simulink model "SimscapeSystemLevel_e8_IPMSM_HWJandVent_ROM"  (R2021b)
settings: Solver=VariableStepAuto  StartTime=0.0  StopTime=300  FixedStep=1  RelTol=1e-3  AbsTol=1e-3
model workspace (MAT data in the model file):
  AdjacencyMat = [0 0 0 0 0 0 0 0 0 0 0 0 ... (15129 elements, 123x123)]
  CapMat = [1e+20 2196.70091586 387.653102799 193.8265514 1962.34710525 387.653102799 193.8265514 1962.34710525 1266.59353814 268.053957132 416.539515956 175.715078 ... (123 elements, 123x1)]
  CoolantArrayIdxs = [20 21 22 23 24 25 26 27 35 36 37 84 ... (19 elements, 19x1)]
  Friction_Loss_Mat = [0 0 0 0 0 0 0 0 0 0 0 0 ... (2340 elements, 39x60)]
  InletCoolIdxs = [37; 38]
  Iron_Loss_Rotor_Back_Iron_Mat = [0.0117705351991 0.0198175800092 0.0246057415963 0.0256631766661 0.0240576767285 0.0207771722396 0.0168311502834 0.0133395315761 0.0115512535049 0.0120779527774 0.0143067244388 0.0171516443454 ... (2340 elements, 39x60)]
  Iron_Loss_Rotor_Pole_Mat = [1.45649756865 1.4525095653 1.42942652973 1.39109338754 1.34251579982 1.287439524 1.22885659237 1.16930852698 1.11098912611 1.05484046499 0.999976047808 0.944563732162 ... (2340 elements, 39x60)]
  Iron_Loss_Rotor_Tooth_Mat = [0 0 0 0 0 0 0 0 0 0 0 0 ... (2340 elements, 39x60)]
  Iron_Loss_Stator_Back_Iron_Mat = [38.5419456951 37.774471759 36.7837540443 35.6885758764 34.5272571596 33.3324529178 32.136302555 30.9744032473 29.8863152048 28.8790573391 27.8876077961 26.8074662049 ... (2340 elements, 39x60)]
  Iron_Loss_Stator_Tooth_Mat = [42.0610884508 41.0604961882 40.1804594162 39.4285940164 38.704339026 37.9602455604 37.1844153901 36.3902226975 35.6050856075 34.8287218867 34.0007237809 33.0439458619 ... (2340 elements, 39x60)]
  LossDistrForEachType = [0 0 0 0 0 0 0 0 0 0 0 0 ... (1968 elements, 16x123)]
  Magnet_Loss_Mat = [0.0995193918038 0.0928899922278 0.0868628846748 0.0818830115456 0.0774722500184 0.0732395922727 0.0687988836096 0.0636930921801 0.0573503948699 0.0496000064543 0.0410757743485 0.0326817704515 ... (2340 elements, 39x60)]
  OutletCoolIdxs = [20; 107]
  ResMat = [0 2.49009256841 6.64572241429 1000000000 1.39790968864 6.64402802995 1000000000 1.39156082742 1000000000 1000000000 1000000000 1000000000 ... (15129 elements, 123x123)]
  RotorCopperTempCoefResistivity = 0.00393
  Rotor_Cage_Loss_Mat = [0 0 0 0 0 0 0 0 0 0 0 0 ... (2340 elements, 39x60)]
  ShaftTorqueVec = [-287.262157301 -272.268610731 -257.275064161 -242.281517591 -227.287971021 -212.294424451 -197.300877881 -182.307331311 -167.31378474 -152.32023817 -137.3266916 -122.33314503 ... (39 elements, 1x39)]
  SpeedVec = [500 661.016949153 822.033898305 983.050847458 1144.06779661 1305.08474576 1466.10169492 1627.11864407 1788.13559322 1949.15254237 2110.16949153 2271.18644068 ... (60 elements, 1x60)]
  StateSpaceND : object (value not decoded)
  StatorCopperTempCoefResistivity = 0.00393
  Stator_Copper_Loss_Mat = [3925.33912093 3510.19452231 3089.33767218 2711.80000483 2370.99356953 2062.06508217 1781.35176729 1526.02799256 1293.87708125 1083.15658499 892.54525431 720.809889245 ... (2340 elements, 39x60)]
  Stray_Load_Loss_Mat = [0 0 0 0 0 0 0 0 0 0 0 0 ... (2340 elements, 39x60)]
  Stray_Loss_Stator_Iron_Proportion = 0.95
  Tgiven = 20
  TnodesInit = [25 25 25 25 25 25 25 25 25 25 25 25 ... (123 elements, 123x1)]
  TrefRotor = 20
  TrefStator = 20
  Windage_Loss_Mat = [0 0 0 0 0 0 0 0 0 0 0 0 ... (2340 elements, 39x60)]
libraries: fl_lib x33, nesl_utility x13, mcadROM_lib x4, simulink_extras x2, autolibshared x1, slpidlib x1, SimscapeFluids_lib x1
(part 2 of 2)

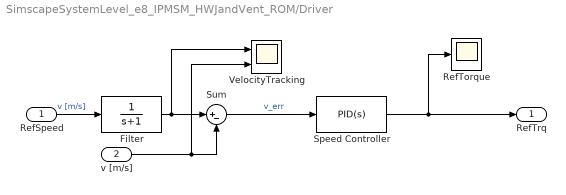
== system SimscapeSystemLevel_e8_IPMSM_HWJandVent_ROM/Driver ==
  RefSpeed : Inport
  v [m/s] : Inport  Port=2
  Filter : TransferFcn  Denominator=[1 1]
  RefTorque : Scope
  Speed Controller : slpidlib/PID Controller  Controller=PID  Form=Parallel  TimeDomain=Continuous-time  UseExternalTs=off  SampleTime=-1  IntegratorMethod=Forward Euler  FilterMethod=Forward Euler  ControllerParametersSource=internal  P=50  I=1e-1  D=0  UseFilter=on  N=100  TunerSelectOption=Transfer Function Based (PID Tuner App)  InitialConditionSource=internal  InitialConditionForIntegrator=0  InitialConditionForFilter=0  DifferentiatorICPrevScaledInput=0  ExternalReset=none  TrackingMode=off  Kt=1  LimitOutput=on  SatLimitsSource=internal  UpperSaturationLimit=150  LowerSaturationLimit=-150  LinearizeAsGain=on  AntiWindupMode=none  Kb=1  POutMin=[]  POutMax=[]  IOutMin=[]  IOutMax=[]  DOutMin=[]  DOutMax=[]  NOutMin=[]  NOutMax=[]  SumOutMin=[]  SumOutMax=[]  SaturationOutMin=[]  SaturationOutMax=[]  PParamMin=[]  PParamMax=[]  IParamMin=[]  IParamMax=[]  DParamMin=[]  DParamMax=[]  NParamMin=[]  NParamMax=[]  KbParamMin=[]  KbParamMax=[]  KtParamMin=[]  KtParamMax=[]  KbOutMin=[]  KbOutMax=[]  KtOutMin=[]  KtOutMax=[]  IntegratorOutMin=[]  IntegratorOutMax=[]  FilterOutMin=[]  FilterOutMax=[]  SumI1OutMin=[]  SumI1OutMax=[]  SumI2OutMin=[]  SumI2OutMax=[]  SumI3OutMin=[]  SumI3OutMax=[]  SumI4OutMin=[]  SumI4OutMax=[]  SumDOutMin=[]  SumDOutMax=[]  DifferentiatorOutMin=[]  DifferentiatorOutMax=[]  FilterDiffOutCoefMin=[]  FilterDiffOutCoefMax=[]  ReciprocalOutMin=[]  ReciprocalOutMax=[]  SumDenOutMin=[]  SumDenOutMax=[]  SumNumOutMin=[]  SumNumOutMax=[]  DivideOutMin=[]  DivideOutMax=[]  UdiffTsProdOutMin=[]  UdiffTsProdOutMax=[]  NTsProdOutMin=[]  NTsProdOutMax=[]  UintegralTsProdOutMin=[]  UintegralTsProdOutMax=[]  UngainTsProdOutMin=[]  UngainTsProdOutMax=[]  FilterDenConstantOutDataTypeStr=Inherit: Inherit via back propagation  FilterDenConstantOutMin=[]  FilterDenConstantOutMax=[]  PCopyOutDataTypeStr=Inherit: Inherit via back propagation  PCopyOutMin=[]  PCopyOutMax=[]  NCopyOutDataTypeStr=Inherit: Inherit via back propagation  NCopyOutMin=[]  NCopyOutMax=[]  IntegratorContinuousStateAttributes=''  IntegratorStateMustResolveToSignalObject=off  IntegratorRTWStateStorageClass=Auto  FilterContinuousStateAttributes=''  FilterStateMustResolveToSignalObject=off  FilterRTWStateStorageClass=Auto  ParallelPVariant=InternalParameters  IdealPVariant=Disabled  IVariant=InternalParameters  DVariant=InternalParameters  IntegratorVariant=Continuous  SatVariant=Enabled  AWVariant=Passthrough  PCopyVariant=Disabled  TRVariant=Disabled  FdbkBlocksVariant=Forward  IdealPFdbkVariant=Disabled  SatFdbkVariant=Disabled  DerivativeFilterVariant=ContFilter  NVariant=InternalParameters  NCopyVariant=Disabled  FilterICVariant=InternalICsFilter  IntegratorICVariant=InternalICs  ExternalResetVariant=Disabled  TRSumVariant=Passthrough  SumFdbkVariant=Disabled  SumVariant=Sum_PID  TsampFilterVariant=InternalTs  TsampNgainVariant=Passthrough  TsampIntegralVariant=Passthrough  ExternalSaturationOutDataTypeStr=Inherit: Same as second input
  Sum : Sum  Inputs=|+-
  VelocityTracking : Scope  NumInputPorts=2
  RefTrq : Outport
  wires:
  v [m/s]/1 -> VelocityTracking/2, Sum/2
  Sum/1 -> Speed Controller/1  "v_err"
  Speed Controller/1 -> RefTorque/1, RefTrq/1
  RefSpeed/1 -> Filter/1  "v [m/s]"
  Filter/1 -> VelocityTracking/1, Sum/1

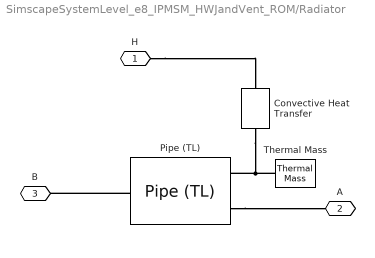
== system SimscapeSystemLevel_e8_IPMSM_HWJandVent_ROM/Radiator ==
  Convective Heat Transfer : fl_lib/Thermal/Thermal Elements/Convective Heat Transfer  area=5 m^2  heat_tr_coeff=20 W/(m^2*K)  T_specify=off  T_priority=None  T=0 K  T_nominal_specify=off  T_nominal_unit=K  T_nominal_value=1  Q_specify=off  Q_priority=None  Q=0 W  Q_nominal_specify=off  Q_nominal_unit=W  Q_nominal_value=1
  Pipe (TL) : fl_lib/Thermal Liquid/Elements/Pipe (TL)  length=5 m  area=0.01 m^2  Dh=0.1128 m  length_add=1 m  roughness=15e-6 m  Re_lam=2000  Re_tur=4000  shape_factor=64  Nu_lam=3.66  dynamic_compressibility=simscape.enum.onoff.on  inertia=simscape.enum.onoff.off  p0=0.101325 MPa  T0=TnodesInit(1) degC  mdot0=0 kg/s
      settings: SourceProductBaseCode=SS
  Thermal Mass : fl_lib/Thermal/Thermal Elements/Thermal Mass  mass=3 kg  sp_heat=447 J/(K*kg)  T_specify=on  T_priority=High  T=TnodesInit(1) degC  T_nominal_specify=off  T_nominal_unit=K  T_nominal_value=1  Q_specify=off  Q_priority=None  Q=0 W  Q_nominal_specify=off  Q_nominal_unit=W  Q_nominal_value=1
  H : PMIOPort  Side=Left
  A : PMIOPort  Port=2  Side=Left
  B : PMIOPort  Port=3  Side=Right
  connections:
  Thermal Mass/LConn1 -- Convective Heat Transfer/LConn1 -- Pipe (TL)/LConn2
  Pipe (TL)/LConn1 -- A/RConn1
  Pipe (TL)/RConn1 -- B/RConn1
  H/RConn1 -- Convective Heat Transfer/RConn1

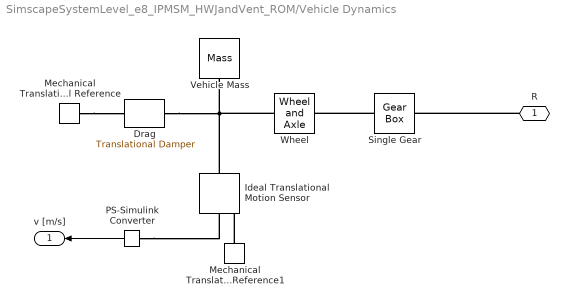
== system SimscapeSystemLevel_e8_IPMSM_HWJandVent_ROM/Vehicle Dynamics ==
  Drag : fl_lib/Mechanical/Translational Elements/Translational Damper  D=25 N/(m/s)  v_specify=off  v_priority=None  v=0 m/s  v_nominal_specify=off  v_nominal_unit=m/s  v_nominal_value=1  f_specify=off  f_priority=None  f=0 N  f_nominal_specify=off  f_nominal_unit=N  f_nominal_value=1
  Ideal Translational Motion Sensor : fl_lib/Mechanical/Mechanical Sensors/Ideal Translational Motion Sensor  offset=0 m
  Mechanical Translational Reference : fl_lib/Mechanical/Translational Elements/Mechanical Translational Reference
  Mechanical Translational Reference1 : fl_lib/Mechanical/Translational Elements/Mechanical Translational Reference
  PS-Simulink Converter : nesl_utility/PS-Simulink Converter  PhysicalDomain=network_engine_domain  SubClassName=ps_output  LeftPortType=input  RightPortType=output  PseudoPeriodic=off  Frequencies=[]  Unit=m/s  AffineConversion=off
      settings: SourceProductBaseCode=PW,SS
  Single Gear : fl_lib/Mechanical/Mechanisms/Gear Box  ratio=1/5  t_in_specify=off  t_in_priority=None  t_in=0 N*m  t_in_nominal_specify=off  t_in_nominal_unit=N*m  t_in_nominal_value=1  t_out_specify=off  t_out_priority=None  t_out=0 N*m  t_out_nominal_specify=off  t_out_nominal_unit=N*m  t_out_nominal_value=1
  Vehicle Mass : fl_lib/Mechanical/Translational Elements/Mass  mass=2000 kg  num_ports=foundation.enum.numPorts2.one  v_specify=off  v_priority=High  v=0 m/s  v_nominal_specify=off  v_nominal_unit=m/s  v_nominal_value=1  f_specify=off  f_priority=None  f=0 N  f_nominal_specify=off  f_nominal_unit=N  f_nominal_value=1
  Wheel : fl_lib/Mechanical/Mechanisms/Wheel and Axle  R=0.15 m  or=1  t_specify=off  t_priority=None  t=0 N*m  t_nominal_specify=off  t_nominal_unit=N*m  t_nominal_value=1  f_specify=off  f_priority=None  f=0 N  f_nominal_specify=off  f_nominal_unit=N  f_nominal_value=1
  R : PMIOPort  Side=Right
  v [m/s] : Outport
  wires:
  PS-Simulink Converter/1 -> v [m/s]/1
  connections:
  R/RConn1 -- Single Gear/RConn1
  Single Gear/LConn1 -- Wheel/LConn1
  Wheel/RConn1 -- Ideal Translational Motion Sensor/LConn1 -- Drag/LConn1 -- Vehicle Mass/LConn1
  Mechanical Translational Reference/LConn1 -- Drag/RConn1
  Mechanical Translational Reference1/LConn1 -- Ideal Translational Motion Sensor/RConn1
  PS-Simulink Converter/LConn1 -- Ideal Translational Motion Sensor/RConn2

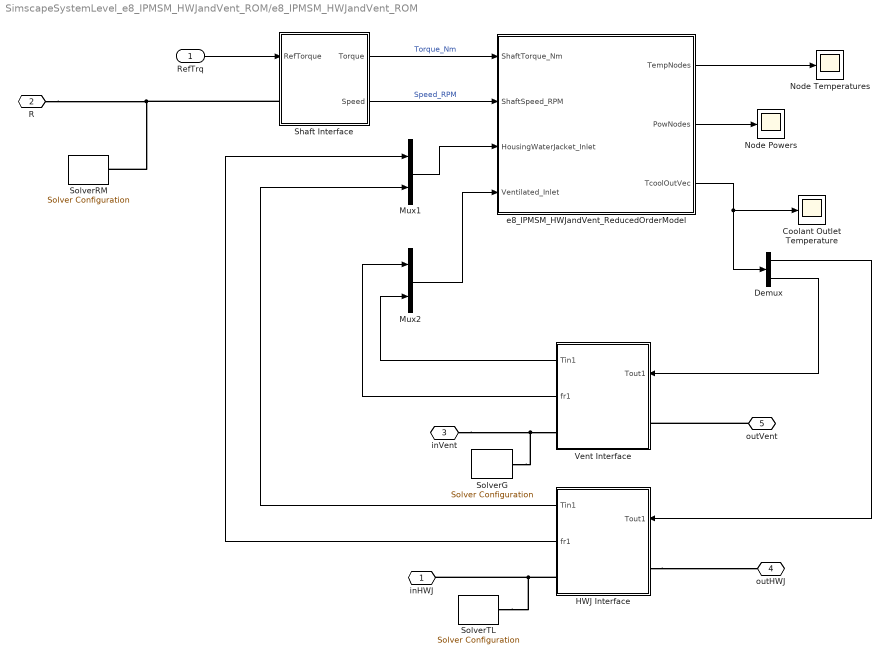
== system SimscapeSystemLevel_e8_IPMSM_HWJandVent_ROM/e8_IPMSM_HWJandVent_ROM ==
  RefTrq : Inport
  Coolant Outlet Temperature : Scope
  Demux : Demux  Outputs=2
  HWJ Interface : Subsystem
      settings: PortSchema="{\"entries\":[{\"content\":{\"sides\":[{\"content\":{\"connectorIds\":[\"Out1\",\"Out2\",\"LConn1\"]},\"type\":\"ConnectorPlacement.EquallySpacedRectSide\",\"uuid\":\"a0734607-c8e3-4baa-99d0-f684b459279a\"},{\"content\":{\"connectorIds\":[\"In1\",\"RConn1\"],\"side\":\"RIGHT\"},\"type\":\"ConnectorPlacement.EquallySpacedRectSide\",\"uuid\":\"b656feb5-3093-4bd9-8bf1-21827cdeeded\"},{\"content\":{\"connectorIds\":[],\"side\":\"TOP\"},\"type\":\"ConnectorPlacement.EquallySpacedRectSide\",\"uuid\":\"2d3f104c-c7aa-4510-969a-a40e5e879ab2\"}]},\"type\":\"ConnectorPlacement.EquallySpacedConnector\",\"uuid\":\"1033d5d5-dd4a-4fd0-a709-c87184322d51\"}],\"packageUris\":[\"http://schema.mathworks.com/mf0/Connector/R2020b\"],\"version\":\"1.0\"}"
  Mux1 : Mux  Inputs=2
  Mux2 : Mux  Inputs=2
  Node Powers : Scope
  Node Temperatures : Scope
  Shaft Interface : Subsystem
  SolverG : nesl_utility/Solver Configuration  PhysicalDomain=network_engine_domain  SubClassName=solver  LeftPortType=input  RightPortType=generic  Tones=[]  Harmonics=[]  SimulateNoise=off  Profile=off  UseLocalSampling=off  EnableSwitchedLinearOptims=on  FrequencyDomain=off  UseCCode=off  RelTol=0.001  AbsTol=1e-06  MinStep=1e-09  ToWorkspace=off  RevertToSquareIcSolve=off  NumHomotopyIterations=100  PhasorMode=off  PhasorModeNumHarmonics=1  DoDC=off  ResidualTolerance=1e-09  UseLocalSolver=off  LocalSolverChoice=NE_BACKWARD_EULER_ADVANCER  LocalSolverSampleTime=0.001  DoFixedCost=off  MaxNonlinIter=3  MaxModeIter=2  ComputeImpulses=off  ImpulseIterations=2  LinearAlgebra=auto  EquationFormulation=NE_TIME_EF  DelaysMemoryBudget=1024  AutomaticFiltering=on  FilteringTimeConstant=0.001  PartitionStorageMethod=AS_NEEDED  PartitionMemoryBudget=1024  PartitionMethod=ROBUST
      settings: SourceProductBaseCode=PW,SS
  SolverRM : nesl_utility/Solver Configuration  PhysicalDomain=network_engine_domain  SubClassName=solver  LeftPortType=input  RightPortType=generic  Tones=[]  Harmonics=[]  SimulateNoise=off  Profile=off  UseLocalSampling=off  EnableSwitchedLinearOptims=on  FrequencyDomain=off  UseCCode=off  RelTol=0.001  AbsTol=1e-06  MinStep=1e-09  ToWorkspace=off  RevertToSquareIcSolve=off  NumHomotopyIterations=100  PhasorMode=off  PhasorModeNumHarmonics=1  DoDC=off  ResidualTolerance=1e-09  UseLocalSolver=off  LocalSolverChoice=NE_BACKWARD_EULER_ADVANCER  LocalSolverSampleTime=0.001  DoFixedCost=off  MaxNonlinIter=3  MaxModeIter=2  ComputeImpulses=off  ImpulseIterations=2  LinearAlgebra=auto  EquationFormulation=NE_TIME_EF  DelaysMemoryBudget=1024  AutomaticFiltering=on  FilteringTimeConstant=0.001  PartitionStorageMethod=AS_NEEDED  PartitionMemoryBudget=1024  PartitionMethod=ROBUST
      settings: SourceProductBaseCode=PW,SS
  SolverTL : nesl_utility/Solver Configuration  PhysicalDomain=network_engine_domain  SubClassName=solver  LeftPortType=input  RightPortType=generic  Tones=[]  Harmonics=[]  SimulateNoise=off  Profile=off  UseLocalSampling=off  EnableSwitchedLinearOptims=on  FrequencyDomain=off  UseCCode=off  RelTol=0.001  AbsTol=1e-06  MinStep=1e-09  ToWorkspace=off  RevertToSquareIcSolve=off  NumHomotopyIterations=100  PhasorMode=off  PhasorModeNumHarmonics=1  DoDC=off  ResidualTolerance=1e-09  UseLocalSolver=off  LocalSolverChoice=NE_BACKWARD_EULER_ADVANCER  LocalSolverSampleTime=0.001  DoFixedCost=off  MaxNonlinIter=3  MaxModeIter=2  ComputeImpulses=off  ImpulseIterations=2  LinearAlgebra=auto  EquationFormulation=NE_TIME_EF  DelaysMemoryBudget=1024  AutomaticFiltering=on  FilteringTimeConstant=0.001  PartitionStorageMethod=AS_NEEDED  PartitionMemoryBudget=1024  PartitionMethod=ROBUST
      settings: SourceProductBaseCode=PW,SS
  Vent Interface : Subsystem
      settings: PortSchema="{\"entries\":[{\"content\":{\"sides\":[{\"content\":{\"connectorIds\":[\"Out1\",\"Out2\",\"LConn1\"]},\"type\":\"ConnectorPlacement.EquallySpacedRectSide\",\"uuid\":\"a0734607-c8e3-4baa-99d0-f684b459279a\"},{\"content\":{\"connectorIds\":[\"In1\",\"RConn1\"],\"side\":\"RIGHT\"},\"type\":\"ConnectorPlacement.EquallySpacedRectSide\",\"uuid\":\"b656feb5-3093-4bd9-8bf1-21827cdeeded\"},{\"content\":{\"connectorIds\":[],\"side\":\"TOP\"},\"type\":\"ConnectorPlacement.EquallySpacedRectSide\",\"uuid\":\"2d3f104c-c7aa-4510-969a-a40e5e879ab2\"}]},\"type\":\"ConnectorPlacement.EquallySpacedConnector\",\"uuid\":\"1033d5d5-dd4a-4fd0-a709-c87184322d51\"}],\"packageUris\":[\"http://schema.mathworks.com/mf0/Connector/R2020b\"],\"version\":\"1.0\"}"
  e8_IPMSM_HWJandVent_ReducedOrderModel : Subsystem
  inHWJ : PMIOPort  Side=Left
  R : PMIOPort  Port=2  Side=Left
  inVent : PMIOPort  Port=3  Side=Left
  outHWJ : PMIOPort  Port=4  Side=Right
  outVent : PMIOPort  Port=5  Side=Right
  wires:
  e8_IPMSM_HWJandVent_ReducedOrderModel/2(PowNodes) -> Node Powers/1
  Mux2/1 -> e8_IPMSM_HWJandVent_ReducedOrderModel/4(Ventilated_Inlet)
  e8_IPMSM_HWJandVent_ReducedOrderModel/1(TempNodes) -> Node Temperatures/1
  Mux1/1 -> e8_IPMSM_HWJandVent_ReducedOrderModel/3(HousingWaterJacket_Inlet)
  e8_IPMSM_HWJandVent_ReducedOrderModel/3(TcoolOutVec) -> Demux/1, Coolant Outlet Temperature/1
  HWJ Interface/2(fr1) -> Mux1/1
  HWJ Interface/1(Tin1) -> Mux1/2
  Demux/1 -> HWJ Interface/1(Tout1)
  Vent Interface/1(Tin1) -> Mux2/2
  Vent Interface/2(fr1) -> Mux2/1
  Demux/2 -> Vent Interface/1(Tout1)
  Shaft Interface/1(Torque) -> e8_IPMSM_HWJandVent_ReducedOrderModel/1(ShaftTorque_Nm)  "Torque_Nm"
  Shaft Interface/2(Speed) -> e8_IPMSM_HWJandVent_ReducedOrderModel/2(ShaftSpeed_RPM)  "Speed_RPM"
  RefTrq/1 -> Shaft Interface/1(RefTorque)
  connections:
  HWJ Interface/RConn1 -- outHWJ/RConn1
  HWJ Interface/LConn1 -- SolverTL/RConn1 -- inHWJ/RConn1
  inVent/RConn1 -- SolverG/RConn1 -- Vent Interface/LConn1
  outVent/RConn1 -- Vent Interface/RConn1
  R/RConn1 -- Shaft Interface/LConn1 -- SolverRM/RConn1

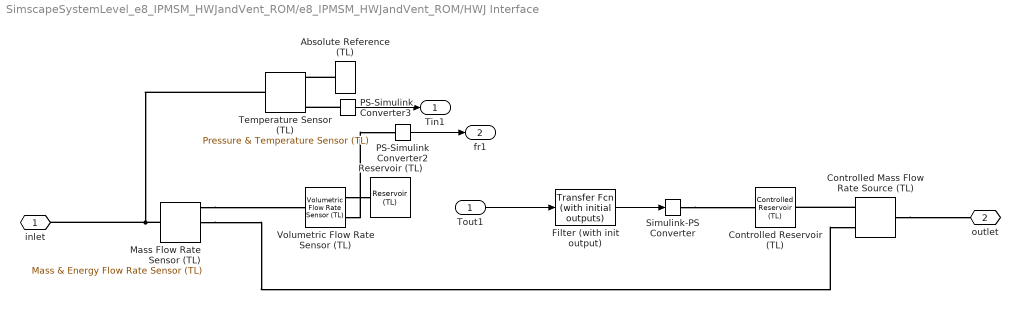
== system SimscapeSystemLevel_e8_IPMSM_HWJandVent_ROM/e8_IPMSM_HWJandVent_ROM/HWJ Interface ==
  Tout1 : Inport
  Absolute Reference (TL) : fl_lib/Thermal Liquid/Elements/Absolute Reference (TL)
      settings: SourceProductBaseCode=SS
  Controlled Mass Flow Rate Source (TL) : fl_lib/Thermal Liquid/Sources/Controlled Mass Flow Rate Source (TL)  area=pi*0.01^2 m^2
      settings: SourceProductBaseCode=SS  InternalSimscapePortConfiguration="{\"Bottom\":[],\"Left\":[{\"id\":\"A\",\"label\":\"A\",\"type\":\"foundation.thermal_liquid.thermal_liquid\"},{\"id\":\"M\",\"label\":\"M\",\"type\":\"input\"}],\"Right\":[{\"id\":\"B\",\"label\":\"B\",\"type\":\"foundation.thermal_liquid.thermal_liquid\"}],\"Top\":[]}"
  Controlled Reservoir (TL) : fl_lib/Thermal Liquid/Elements/Controlled Reservoir (TL)  pressure_spec=foundation.enum.pressure_spec.specified  reservoir_pressure=0.101325 MPa  area=pi*0.01^2 m^2
      settings: SourceProductBaseCode=SS  InternalSimscapePortConfiguration="{\"Bottom\":[],\"Left\":[{\"id\":\"A\",\"label\":\"A\",\"type\":\"foundation.thermal_liquid.thermal_liquid\"}],\"Right\":[{\"id\":\"T_in\",\"label\":\"T\",\"type\":\"input\"}],\"Top\":[]}"
  Filter (with init output) : simulink_extras/Additional Linear/Transfer Fcn (with initial outputs)  N=[1]  D="[1  1]"  Y0=.5  U0=TnodesInit(1)
  Mass Flow Rate Sensor (TL) : fl_lib/Thermal Liquid/Sensors/Mass & Energy Flow Rate Sensor (TL)
      settings: SourceProductBaseCode=SS  InternalSimscapePortConfiguration="{\"Bottom\":[],\"Left\":[{\"id\":\"A\",\"label\":\"A\",\"type\":\"foundation.thermal_liquid.thermal_liquid\"}],\"Right\":[{\"id\":\"B\",\"label\":\"B\",\"type\":\"foundation.thermal_liquid.thermal_liquid\"},{\"id\":\"M\",\"label\":\"M\",\"type\":\"output\"},{\"id\":\"PHI\",\"label\":\"Phi\",\"type\":\"output\"}],\"Top\":[]}"
  PS-Simulink Converter2 : nesl_utility/PS-Simulink Converter  PhysicalDomain=network_engine_domain  SubClassName=ps_output  LeftPortType=input  RightPortType=output  PseudoPeriodic=off  Frequencies=[]  Unit=lpm  AffineConversion=off
      settings: SourceProductBaseCode=PW,SS
  PS-Simulink Converter3 : nesl_utility/PS-Simulink Converter  PhysicalDomain=network_engine_domain  SubClassName=ps_output  LeftPortType=input  RightPortType=output  PseudoPeriodic=off  Frequencies=[]  Unit=degC  AffineConversion=on
      settings: SourceProductBaseCode=PW,SS
  Reservoir (TL) : fl_lib/Thermal Liquid/Elements/Reservoir (TL)  pressure_spec=foundation.enum.pressure_spec.specified  reservoir_pressure=0.101325 MPa  reservoir_temperature=TnodesInit(1) degC  area=pi*0.01^2 m^2
      settings: SourceProductBaseCode=SS
  Simulink-PS Converter : nesl_utility/Simulink-PS Converter  PhysicalDomain=network_engine_domain  SubClassName=ps_input  LeftPortType=input  RightPortType=output  PseudoPeriodic=off  Frequencies=[]  NoiseDistribution=none  NoiseParameters=[]  Unit=degC  AffineConversion=on  FilteringAndDerivatives=provide  SimscapeFilterOrder=1  InputFilterTimeConstant=0.001  UdotUserProvided=0
      settings: SourceProductBaseCode=PW,SS
  Temperature Sensor (TL) : fl_lib/Thermal Liquid/Sensors/Pressure & Temperature Sensor (TL)
      settings: SourceProductBaseCode=SS  InternalSimscapePortConfiguration="{\"Bottom\":[],\"Left\":[{\"id\":\"A\",\"label\":\"A\",\"type\":\"foundation.thermal_liquid.thermal_liquid\"}],\"Right\":[{\"id\":\"B\",\"label\":\"B\",\"type\":\"foundation.thermal_liquid.thermal_liquid\"},{\"id\":\"P\",\"label\":\"P\",\"type\":\"output\"},{\"id\":\"T\",\"label\":\"T\",\"type\":\"output\"}],\"Top\":[]}"
  Volumetric Flow Rate Sensor (TL) : fl_lib/Thermal Liquid/Sensors/Volumetric Flow Rate Sensor (TL)
      settings: SourceProductBaseCode=SS  InternalSimscapePortConfiguration="{\"Bottom\":[],\"Left\":[{\"id\":\"A\",\"label\":\"A\",\"type\":\"foundation.thermal_liquid.thermal_liquid\"}],\"Right\":[{\"id\":\"B\",\"label\":\"B\",\"type\":\"foundation.thermal_liquid.thermal_liquid\"},{\"id\":\"V\",\"label\":\"V\",\"type\":\"output\"}],\"Top\":[]}"
  inlet : PMIOPort  Side=Left
  outlet : PMIOPort  Port=2  Side=Right
  Tin1 : Outport
  fr1 : Outport  Port=2
  wires:
  PS-Simulink Converter2/1 -> fr1/1
  PS-Simulink Converter3/1 -> Tin1/1
  Filter (with init output)/1 -> Simulink-PS Converter/1
  Tout1/1 -> Filter (with init output)/1
  connections:
  Volumetric Flow Rate Sensor (TL)/RConn1 -- Reservoir (TL)/LConn1
  PS-Simulink Converter3/LConn1 -- Temperature Sensor (TL)/RConn3
  Volumetric Flow Rate Sensor (TL)/RConn2 -- PS-Simulink Converter2/LConn1
  Controlled Mass Flow Rate Source (TL)/LConn1 -- Controlled Reservoir (TL)/LConn1
  Mass Flow Rate Sensor (TL)/LConn1 -- inlet/RConn1 -- Temperature Sensor (TL)/LConn1
  Absolute Reference (TL)/LConn1 -- Temperature Sensor (TL)/RConn1
  Mass Flow Rate Sensor (TL)/RConn1 -- Volumetric Flow Rate Sensor (TL)/LConn1
  Mass Flow Rate Sensor (TL)/RConn2 -- Controlled Mass Flow Rate Source (TL)/LConn2
  Simulink-PS Converter/RConn1 -- Controlled Reservoir (TL)/RConn1
  Controlled Mass Flow Rate Source (TL)/RConn1 -- outlet/RConn1

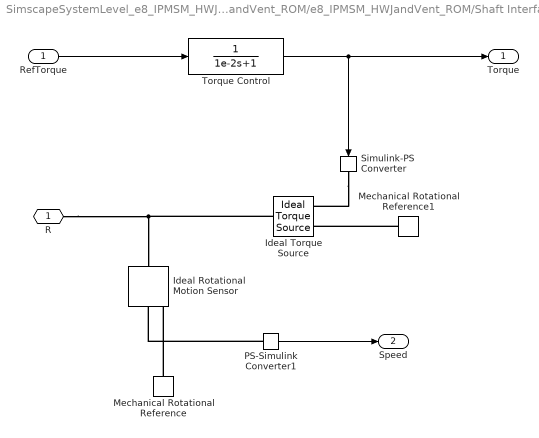
== system SimscapeSystemLevel_e8_IPMSM_HWJandVent_ROM/e8_IPMSM_HWJandVent_ROM/Shaft Interface ==
  RefTorque : Inport
  Ideal Rotational Motion Sensor : fl_lib/Mechanical/Mechanical Sensors/Ideal Rotational Motion Sensor  wrap_angle=simscape.enum.onoff.off  offset=0 rad
  Ideal Torque Source : fl_lib/Mechanical/Mechanical Sources/Ideal Torque Source
  Mechanical Rotational Reference : fl_lib/Mechanical/Rotational Elements/Mechanical Rotational Reference
  Mechanical Rotational Reference1 : fl_lib/Mechanical/Rotational Elements/Mechanical Rotational Reference
  PS-Simulink Converter1 : nesl_utility/PS-Simulink Converter  PhysicalDomain=network_engine_domain  SubClassName=ps_output  LeftPortType=input  RightPortType=output  PseudoPeriodic=off  Frequencies=[]  Unit=rpm  AffineConversion=off
      settings: SourceProductBaseCode=PW,SS
  Simulink-PS Converter : nesl_utility/Simulink-PS Converter  PhysicalDomain=network_engine_domain  SubClassName=ps_input  LeftPortType=input  RightPortType=output  PseudoPeriodic=off  Frequencies=[]  NoiseDistribution=none  NoiseParameters=[]  Unit=N*m  AffineConversion=off  FilteringAndDerivatives=provide  SimscapeFilterOrder=1  InputFilterTimeConstant=0.001  UdotUserProvided=0
      settings: SourceProductBaseCode=PW,SS
  Torque Control : TransferFcn  Denominator=[1e-2 1]
  R : PMIOPort  Side=Left
  Torque : Outport
  Speed : Outport  Port=2
  wires:
  PS-Simulink Converter1/1 -> Speed/1
  RefTorque/1 -> Torque Control/1
  Torque Control/1 -> Torque/1, Simulink-PS Converter/1
  connections:
  R/RConn1 -- Ideal Torque Source/LConn1 -- Ideal Rotational Motion Sensor/LConn1
  Mechanical Rotational Reference/LConn1 -- Ideal Rotational Motion Sensor/RConn1
  PS-Simulink Converter1/LConn1 -- Ideal Rotational Motion Sensor/RConn2
  Mechanical Rotational Reference1/LConn1 -- Ideal Torque Source/RConn2
  Simulink-PS Converter/RConn1 -- Ideal Torque Source/RConn1

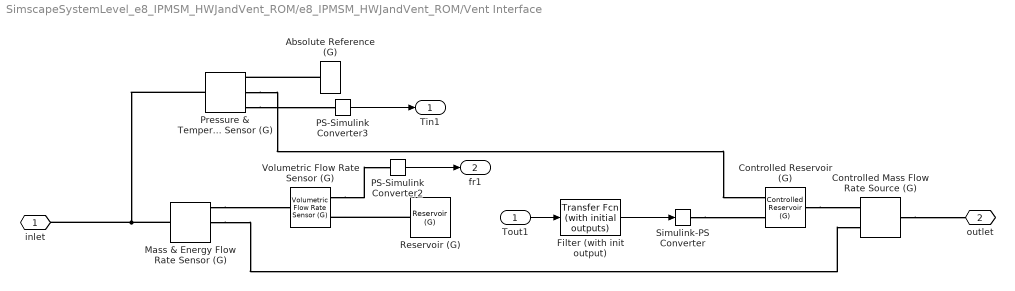
== system SimscapeSystemLevel_e8_IPMSM_HWJandVent_ROM/e8_IPMSM_HWJandVent_ROM/Vent Interface ==
  Tout1 : Inport
  Absolute Reference (G) : fl_lib/Gas/Elements/Absolute Reference (G)
      settings: SourceProductBaseCode=SS  InternalSimscapePortConfiguration="{\"Bottom\":[],\"Left\":[{\"id\":\"A\",\"label\":\"\",\"type\":\"foundation.gas.gas\"}],\"Right\":[],\"Top\":[]}"
  Controlled Mass Flow Rate Source (G) : fl_lib/Gas/Sources/Controlled Mass Flow Rate Source (G)  power_spec=foundation.enum.power_spec.isentropic  area_A=0.01 m^2  area_B=0.01 m^2
      settings: SourceProductBaseCode=SS  InternalSimscapePortConfiguration="{\"Bottom\":[],\"Left\":[{\"id\":\"A\",\"label\":\"A\",\"type\":\"foundation.gas.gas\"},{\"id\":\"M\",\"label\":\"M\",\"type\":\"input\"}],\"Right\":[{\"id\":\"B\",\"label\":\"B\",\"type\":\"foundation.gas.gas\"}],\"Top\":[]}"
  Controlled Reservoir (G) : fl_lib/Gas/Elements/Controlled Reservoir (G)  area_A=0.01 m^2
      settings: SourceProductBaseCode=SS  InternalSimscapePortConfiguration="{\"Bottom\":[],\"Left\":[{\"id\":\"A\",\"label\":\"A\",\"type\":\"foundation.gas.gas\"}],\"Right\":[{\"id\":\"T_in\",\"label\":\"T\",\"type\":\"input\"},{\"id\":\"p_in\",\"label\":\"P\",\"type\":\"input\"}],\"Top\":[]}"
  Filter (with init output) : simulink_extras/Additional Linear/Transfer Fcn (with initial outputs)  N=[1]  D="[1  1]"  Y0=.5  U0=TnodesInit(1)
  Mass & Energy Flow Rate Sensor (G) : fl_lib/Gas/Sensors/Mass & Energy Flow Rate Sensor (G)
      settings: SourceProductBaseCode=SS  InternalSimscapePortConfiguration="{\"Bottom\":[],\"Left\":[{\"id\":\"A\",\"label\":\"A\",\"type\":\"foundation.gas.gas\"}],\"Right\":[{\"id\":\"B\",\"label\":\"B\",\"type\":\"foundation.gas.gas\"},{\"id\":\"M\",\"label\":\"M\",\"type\":\"output\"},{\"id\":\"PHI\",\"label\":\"Phi\",\"type\":\"output\"}],\"Top\":[]}"
  PS-Simulink Converter2 : nesl_utility/PS-Simulink Converter  PhysicalDomain=network_engine_domain  SubClassName=ps_output  LeftPortType=input  RightPortType=output  PseudoPeriodic=off  Frequencies=[]  Unit=lpm  AffineConversion=off
      settings: SourceProductBaseCode=PW,SS
  PS-Simulink Converter3 : nesl_utility/PS-Simulink Converter  PhysicalDomain=network_engine_domain  SubClassName=ps_output  LeftPortType=input  RightPortType=output  PseudoPeriodic=off  Frequencies=[]  Unit=degC  AffineConversion=on
      settings: SourceProductBaseCode=PW,SS
  Pressure & Temperature Sensor (G) : fl_lib/Gas/Sensors/Pressure & Temperature Sensor (G)
      settings: SourceProductBaseCode=SS  InternalSimscapePortConfiguration="{\"Bottom\":[],\"Left\":[{\"id\":\"A\",\"label\":\"A\",\"type\":\"foundation.gas.gas\"}],\"Right\":[{\"id\":\"B\",\"label\":\"B\",\"type\":\"foundation.gas.gas\"},{\"id\":\"P\",\"label\":\"P\",\"type\":\"output\"},{\"id\":\"T\",\"label\":\"T\",\"type\":\"output\"}],\"Top\":[]}"
  Reservoir (G) : fl_lib/Gas/Elements/Reservoir (G)  pressure_spec=foundation.enum.pressure_spec.specified  reservoir_pressure=0.101325 MPa  reservoir_temperature=TnodesInit(1) degC  area_A=0.01 m^2
      settings: SourceProductBaseCode=SS
  Simulink-PS Converter : nesl_utility/Simulink-PS Converter  PhysicalDomain=network_engine_domain  SubClassName=ps_input  LeftPortType=input  RightPortType=output  PseudoPeriodic=off  Frequencies=[]  NoiseDistribution=none  NoiseParameters=[]  Unit=degC  AffineConversion=on  FilteringAndDerivatives=provide  SimscapeFilterOrder=1  InputFilterTimeConstant=0.001  UdotUserProvided=0
      settings: SourceProductBaseCode=PW,SS
  Volumetric Flow Rate Sensor (G) : fl_lib/Gas/Sensors/Volumetric Flow Rate Sensor (G)
      settings: SourceProductBaseCode=SS  InternalSimscapePortConfiguration="{\"Bottom\":[],\"Left\":[{\"id\":\"A\",\"label\":\"A\",\"type\":\"foundation.gas.gas\"}],\"Right\":[{\"id\":\"B\",\"label\":\"B\",\"type\":\"foundation.gas.gas\"},{\"id\":\"V\",\"label\":\"V\",\"type\":\"output\"}],\"Top\":[]}"
  inlet : PMIOPort  Side=Left
  outlet : PMIOPort  Port=2  Side=Right
  Tin1 : Outport
  fr1 : Outport  Port=2
  wires:
  PS-Simulink Converter2/1 -> fr1/1
  PS-Simulink Converter3/1 -> Tin1/1
  Filter (with init output)/1 -> Simulink-PS Converter/1
  Tout1/1 -> Filter (with init output)/1
  connections:
  Pressure & Temperature Sensor (G)/RConn3 -- PS-Simulink Converter3/LConn1
  Volumetric Flow Rate Sensor (G)/RConn2 -- PS-Simulink Converter2/LConn1
  Pressure & Temperature Sensor (G)/LConn1 -- Mass & Energy Flow Rate Sensor (G)/LConn1 -- inlet/RConn1
  Simulink-PS Converter/RConn1 -- Controlled Reservoir (G)/RConn1
  Reservoir (G)/LConn1 -- Volumetric Flow Rate Sensor (G)/RConn1
  Absolute Reference (G)/LConn1 -- Pressure & Temperature Sensor (G)/RConn1
  Pressure & Temperature Sensor (G)/RConn2 -- Controlled Reservoir (G)/RConn2
  Controlled Mass Flow Rate Source (G)/RConn1 -- outlet/RConn1
  Controlled Reservoir (G)/LConn1 -- Controlled Mass Flow Rate Source (G)/LConn1
  Mass & Energy Flow Rate Sensor (G)/RConn1 -- Volumetric Flow Rate Sensor (G)/LConn1
  Mass & Energy Flow Rate Sensor (G)/RConn2 -- Controlled Mass Flow Rate Source (G)/LConn2

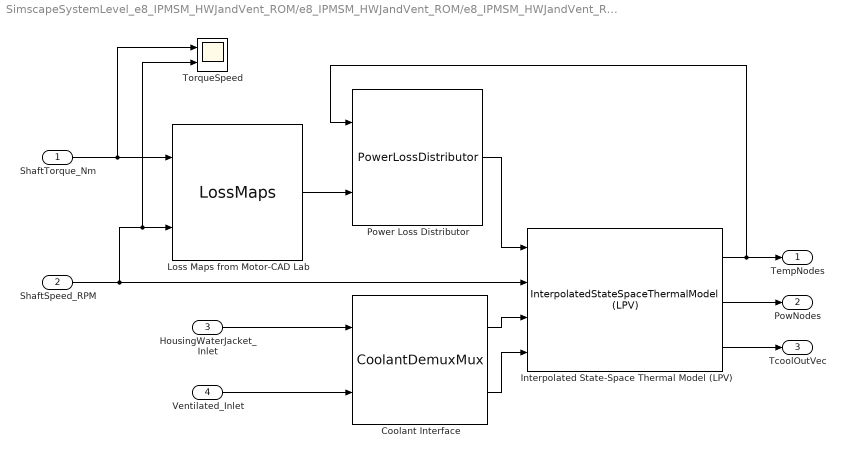
== system SimscapeSystemLevel_e8_IPMSM_HWJandVent_ROM/e8_IPMSM_HWJandVent_ROM/e8_IPMSM_HWJandVent_ReducedOrderModel ==
  ShaftTorque_Nm : Inport
  ShaftSpeed_RPM : Inport  Port=2
  HousingWaterJacket_Inlet : Inport  Port=3
  Ventilated_Inlet : Inport  Port=4
  Coolant Interface : mcadROM_lib/CoolantDemuxMux  numCoolSys=2
  Interpolated State-Space Thermal Model (LPV) : mcadROM_lib/InterpolatedStateSpaceThermalModel (LPV)  StateSpaceND=StateSpaceND  CoolAdjMat=AdjacencyMat  CoolantArrayIdxs=CoolantArrayIdxs  InletCoolantIdxs=InletCoolIdxs  OutletCoolantIdxs=OutletCoolIdxs  TnodesInit=TnodesInit
  Loss Maps from Motor-CAD Lab : mcadROM_lib/LossMaps  ShaftTorqueVec=ShaftTorqueVec  SpeedVec=SpeedVec  Stator_Copper_Loss_Mat=Stator_Copper_Loss_Mat  Rotor_Cage_Loss_Mat=Rotor_Cage_Loss_Mat  Iron_Loss_Stator_Back_Iron_Mat=Iron_Loss_Stator_Back_Iron_Mat  Iron_Loss_Stator_Tooth_Mat=Iron_Loss_Stator_Tooth_Mat  Stray_Loss_Stator_Iron_Proportion=Stray_Loss_Stator_Iron_Proportion  Stray_Load_Loss_Mat=Stray_Load_Loss_Mat  Magnet_Loss_Mat=Magnet_Loss_Mat  Iron_Loss_Rotor_Pole_Mat=Iron_Loss_Rotor_Pole_Mat  Iron_Loss_Rotor_Back_Iron_Mat=Iron_Loss_Rotor_Back_Iron_Mat  Iron_Loss_Rotor_Tooth_Mat=Iron_Loss_Rotor_Tooth_Mat  Friction_Loss_Mat=Friction_Loss_Mat  Windage_Loss_Mat=Windage_Loss_Mat
  Power Loss Distributor : mcadROM_lib/PowerLossDistributor  TrefStator=20  StatorCopperTempCoefResistivity=StatorCopperTempCoefResistivity  TrefRotor=20  RotorCopperTempCoefResistivity=1e-5  LossDistrForEachType=LossDistrForEachType  CapMat=CapMat  CoolantArrayIdxs=CoolantArrayIdxs
  TorqueSpeed : Scope  NumInputPorts=2
  TempNodes : Outport
  PowNodes : Outport  Port=2
  TcoolOutVec : Outport  Port=3
  wires:
  Interpolated State-Space Thermal Model (LPV)/1 -> Power Loss Distributor/1, TempNodes/1
  HousingWaterJacket_Inlet/1 -> Coolant Interface/1
  Interpolated State-Space Thermal Model (LPV)/3 -> TcoolOutVec/1
  Loss Maps from Motor-CAD Lab/1 -> Power Loss Distributor/2
  Coolant Interface/1 -> Interpolated State-Space Thermal Model (LPV)/3
  Ventilated_Inlet/1 -> Coolant Interface/2
  ShaftTorque_Nm/1 -> TorqueSpeed/1, Loss Maps from Motor-CAD Lab/1
  Coolant Interface/2 -> Interpolated State-Space Thermal Model (LPV)/4
  Interpolated State-Space Thermal Model (LPV)/2 -> PowNodes/1
  ShaftSpeed_RPM/1 -> Interpolated State-Space Thermal Model (LPV)/2, TorqueSpeed/2, Loss Maps from Motor-CAD Lab/2
  Power Loss Distributor/1 -> Interpolated State-Space Thermal Model (LPV)/1
